simulink model "verfugarer"  (R2019b)
settings: Solver=VariableStepAuto  StartTime=0.0  StopTime=10.0  RelTol=1e-3
libraries: fl_lib x12
settings Model: Creator=ga  LastModifiedBy=ga

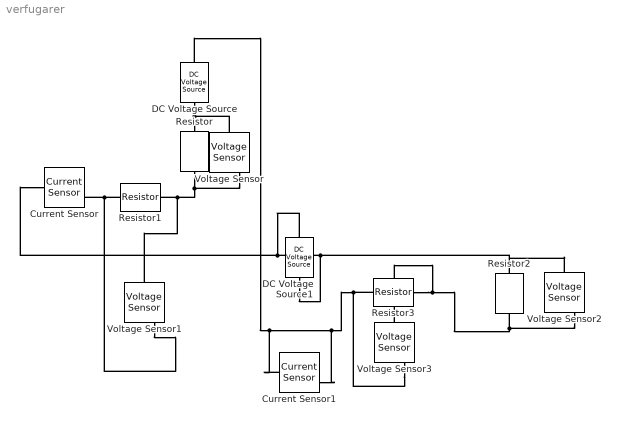
== system verfugarer ==
  Current Sensor : fl_lib/Electrical/Electrical Sensors/Current Sensor
  Current Sensor1 : fl_lib/Electrical/Electrical Sensors/Current Sensor
  DC Voltage Source : fl_lib/Electrical/Electrical Sources/DC Voltage Source  v0=1 V
  DC Voltage Source1 : fl_lib/Electrical/Electrical Sources/DC Voltage Source  v0=1 V
  Resistor{,1..3} (4 alike) : fl_lib/Electrical/Electrical Elements/Resistor  R=1 Ohm  i_specify=off  i_priority=None  i=0 A  i_nominal_specify=off  i_nominal_unit=A  i_nominal_value=1  v_specify=off  v_priority=None  v=0 V  v_nominal_specify=off  v_nominal_unit=V  v_nominal_value=1
  Voltage Sensor{,1..3} (4 alike) : fl_lib/Electrical/Electrical Sensors/Voltage Sensor
  connections:
  Resistor/RConn1 -- Voltage Sensor/RConn2 -- Voltage Sensor1/LConn1 -- Resistor1/RConn1
  DC Voltage Source/LConn1 -- Current Sensor1/LConn1 -- Current Sensor1/RConn2 -- Voltage Sensor3/RConn2 -- Resistor3/LConn1
  DC Voltage Source/RConn1 -- Voltage Sensor/LConn1 -- Resistor/LConn1
  Resistor1/LConn1 -- Voltage Sensor1/RConn2 -- Current Sensor/RConn2
  DC Voltage Source1/RConn1 -- Current Sensor/LConn1 -- DC Voltage Source1/LConn1 -- Voltage Sensor2/LConn1 -- Resistor2/LConn1
  Resistor3/RConn1 -- Voltage Sensor3/LConn1 -- Voltage Sensor2/RConn2 -- Resistor2/RConn1
